simulink model "SRM"  (R2020a)
settings: Solver=VariableStepAuto  StartTime=0.0  StopTime=1  RelTol=1e-3
undefined symbols (not defined in the file): DiscIntNeverNeededParam, Ion, Lithium, Ts
libraries: powerlib x14, electricdrivelib x1
settings Model: Creator=Toan Thanh Nguyen  LastModifiedBy=NIKHIL
settings SFSimCC: CustomCodeUndefinedFunction=UseInterfaceOnly

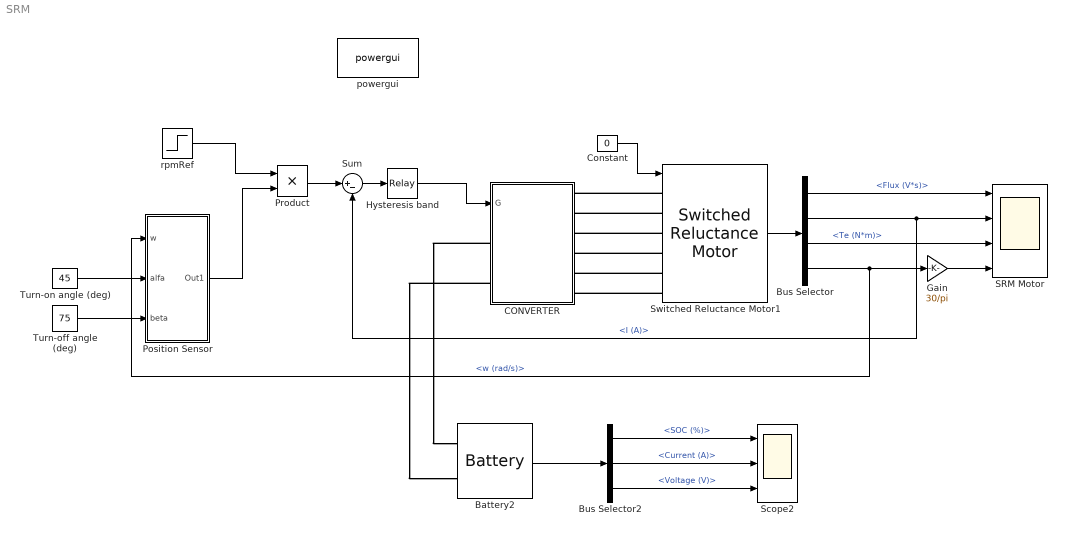
== system SRM ==
  Battery2 : electricdrivelib/Extra Sources/Battery  BatType=Lithium-Ion  ShowTempParam=off  ThermalPreset=no  ShowAgeParam=off  NomV=240  NomQ=5.4  SOC=100  Batt_Tr=30  PresetModel=on  MaxQ=5.4  MinV=180  FullV=279.3569  Dis_rate=2.3478  R=0.44444  Normal_OP=4.8835  expZone="[259.2926     0.2653043]"  current=[6.5 13 32.5]  Units=Time  Tci=20  NomT=20  T2=-30  MaxQ2=4.8  FullV2=7.1  Normal_OP2=5.655  expZone2="[6.58           1]"  Rca=0.6  ti=2000  Dp=0  Neq0=0  Tsim=1e6  Ta1=25  Qeol=5.4*0.9  Reol=0.013333*1.2  Char_age=[2.3478, 3]  Dis_age=[2.3478, 10]  N1=1500  N2=10500  N3=1000  N4=1400  Ta2=45  N5=950
  Bus Selector : BusSelector  OutputSignals=Flux (V*s),I (A),Te (N*m),w (rad/s)
  Bus Selector2 : BusSelector  OutputSignals=SOC (%),Current (A),Voltage (V)
  CONVERTER : Subsystem
  Constant : Constant  Value=0
  Gain : Gain  Gain=30/pi
  "Hysteresis band " : Relay  OnSwitchValue=10  OffSwitchValue=-10
  Position Sensor : Subsystem
  Product : Product
  SRM Motor : Scope  NumInputPorts=4
  Scope2 : Scope  NumInputPorts=3
  Sum : Sum  Inputs=|+-
  Switched Reluctance Motor1 : powerlib/Machines/Switched Reluctance Motor  MachineType=6/4  StatorResistance=0.05  Inertia=0.05  Friction=0.02  InitialSpeed=[0 0]  TsPowergui=0  TsBlock=Ts  MachineModel=Specific model  Lq=0.67e-3  Ld=23.6e-3  Lsat=0.15e-3  MaximumCurrent=450  MaximumFluxLinkage=0.486  Source=MAT-file  MagnetisationCharacteristic='srm64_60kw.mat'  RotorAngleVector=[0 10 20 30 40 45]  StatorCurrentVector=[0:25:450]  PlotCurves=off
      settings: SourceProductBaseCode=PS
  "Turn-off angle (deg) " : Constant  Value=75
  "Turn-on angle (deg) " : Constant  Value=45
  powergui : powerlib/powergui  Priority=1  SimulationMode=Discrete  SampleTime=1e-06  frequency=60  Iterations=50  frequencyindice=0  Pbase=100e6  ErrMax=1e-4  UnitsV=kV  UnitsW=MW  buscounter=0  FunctionMessages=off  echomessages=off  EnableUseOfTLC=off  CurrentSourceSwitches=off  DisableSnubberDevices=off  DisableRonSwitches=off  DisableVfSwitches=off  DisplayEquations=off  AutomaticDiscreteSolvers=off  SolverType=Tustin/Backward Euler (TBE)  Interpol=off  ExternalGateDelay=off  methode=off  Ts=100  x0status=blocks  SPID=on  SwTol=0  HookPort=off  NonlinearTolerance=0  nMaxIteration=15  ContinueOnMaxIteration=off  RestoreLinks=warning  ResistiveCurrentMeasurement=off  Frange=[0:2:500]  Ylog=off  Xlog=on  ShowGrid=off  save=off  variable=ZData  structure=0  ZoomFFT=off  StartTime=0.0  cycles=1  DisplayStyle=1  fundamental=60  FreqAxis=off  MaxFrequency=1000  frequencyindicesteady=1  RmsSteady=1  display=off
  rpmRef : Step  Time=0.1  Before=500  After=0  SampleTime=0
  wires:
  Constant/1 -> Switched Reluctance Motor1/1
  "Hysteresis band "/1 -> CONVERTER/1(G)
  Switched Reluctance Motor1/1 -> Bus Selector/1
  Bus Selector/4 -> Position Sensor/1(w), Gain/1  "<w (rad/s)>"
  Bus Selector/3 -> SRM Motor/3  "<Te (N*m)>"
  Bus Selector/2 -> Sum/2, SRM Motor/2  "<I (A)>"
  Bus Selector/1 -> SRM Motor/1  "<Flux (V*s)>"
  "Turn-on angle (deg) "/1 -> Position Sensor/2(alfa)
  "Turn-off angle (deg) "/1 -> Position Sensor/3(beta)
  Position Sensor/1(Out1) -> Product/2
  Product/1 -> Sum/1
  Sum/1 -> "Hysteresis band "/1
  Gain/1 -> SRM Motor/4
  rpmRef/1 -> Product/1
  Bus Selector2/2 -> Scope2/2  "<Current (A)>"
  Battery2/1 -> Bus Selector2/1
  Bus Selector2/1 -> Scope2/1  "<SOC (%)>"
  Bus Selector2/3 -> Scope2/3  "<Voltage (V)>"
  connections:
  Switched Reluctance Motor1/LConn6 -- CONVERTER/RConn6
  Switched Reluctance Motor1/LConn5 -- CONVERTER/RConn5
  Switched Reluctance Motor1/LConn4 -- CONVERTER/RConn4
  Switched Reluctance Motor1/LConn3 -- CONVERTER/RConn3
  Switched Reluctance Motor1/LConn2 -- CONVERTER/RConn2
  Switched Reluctance Motor1/LConn1 -- CONVERTER/RConn1
  CONVERTER/LConn1 -- Battery2/LConn1
  CONVERTER/LConn2 -- Battery2/LConn2

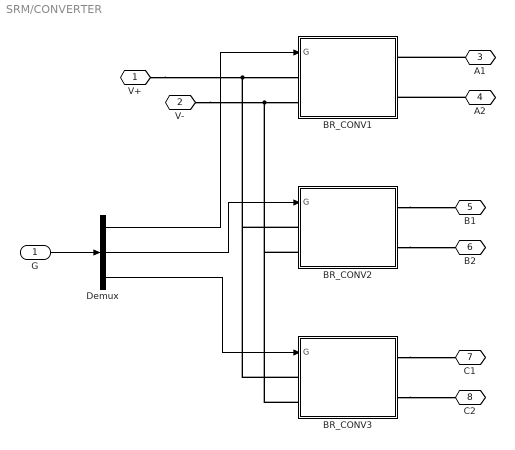
== system SRM/CONVERTER ==
  G : Inport
  BR_CONV1 : Subsystem
  BR_CONV2 : Subsystem
  BR_CONV3 : Subsystem
  Demux : Demux  Outputs=3
  V+ : PMIOPort  Side=Left
  V- : PMIOPort  Port=2  Side=Left
  A1 : PMIOPort  Port=3  Side=Right
  A2 : PMIOPort  Port=4  Side=Right
  B1 : PMIOPort  Port=5  Side=Right
  B2 : PMIOPort  Port=6  Side=Right
  C1 : PMIOPort  Port=7  Side=Right
  C2 : PMIOPort  Port=8  Side=Right
  wires:
  G/1 -> Demux/1
  Demux/1 -> BR_CONV1/1(G)
  Demux/2 -> BR_CONV2/1(G)
  Demux/3 -> BR_CONV3/1(G)
  connections:
  V-/RConn1 -- BR_CONV3/LConn2 -- BR_CONV2/LConn2 -- BR_CONV1/LConn2
  V+/RConn1 -- BR_CONV3/LConn1 -- BR_CONV2/LConn1 -- BR_CONV1/LConn1
  A1/RConn1 -- BR_CONV1/RConn1
  A2/RConn1 -- BR_CONV1/RConn2
  BR_CONV2/RConn1 -- B1/RConn1
  BR_CONV2/RConn2 -- B2/RConn1
  BR_CONV3/RConn1 -- C1/RConn1
  BR_CONV3/RConn2 -- C2/RConn1

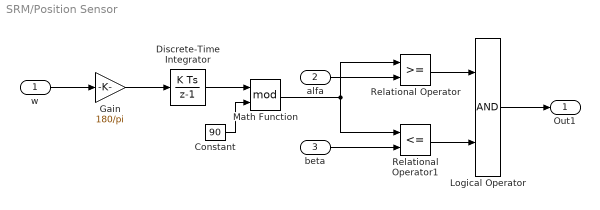
== system SRM/Position Sensor ==
  w : Inport
  alfa : Inport  Port=2
  beta : Inport  Port=3
  Constant : Constant  Value=90
  Discrete-Time Integrator : DiscreteIntegrator  InitialCondition=[0 -30 -60]  SampleTime=Ts  ICPrevOutput=DiscIntNeverNeededParam  ICPrevScaledInput=DiscIntNeverNeededParam
  Gain : Gain  Gain=180/pi
  Logical Operator : Logic  AllPortsSameDT=off  OutDataTypeStr=boolean
  Math Function : Math  Operator=mod  SignedPower=on  SaturateOnIntegerOverflow=on
  Relational Operator : RelationalOperator  OutDataTypeStr=boolean  RndMeth=Simplest
  Relational Operator1 : RelationalOperator  Operator=<=  OutDataTypeStr=boolean  RndMeth=Simplest
  Out1 : Outport  VectorParamsAs1DForOutWhenUnconnected=off
  wires:
  w/1 -> Gain/1
  Gain/1 -> Discrete-Time Integrator/1
  Discrete-Time Integrator/1 -> Math Function/1
  Constant/1 -> Math Function/2
  Math Function/1 -> Relational Operator/1, Relational Operator1/1
  alfa/1 -> Relational Operator/2
  beta/1 -> Relational Operator1/2
  Relational Operator/1 -> Logical Operator/1
  Relational Operator1/1 -> Logical Operator/2
  Logical Operator/1 -> Out1/1

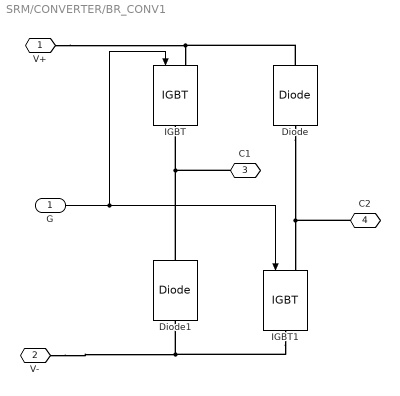
== system SRM/CONVERTER/BR_CONV1 ==
  G : Inport
  Diode : powerlib/Power Electronics/Diode  Ron=1E-3  Lon=0  Vf=0.8  IC=0  UseSnubber=0  Rs=1000  Cs=inf  Measurements=off
  Diode1 : powerlib/Power Electronics/Diode  Ron=1E-3  Lon=0  Vf=0.8  IC=0  UseSnubber=0  Rs=1000  Cs=inf  Measurements=off
  IGBT : powerlib/Power Electronics/IGBT  Ron=1E-3  Lon=0  Vf=1  Tf=1e-6  Tt=2e-6  IC=0  Rs=200  Cs=0.1E-06  Measurements=off
  IGBT1 : powerlib/Power Electronics/IGBT  Ron=1E-3  Lon=0  Vf=1  Tf=1e-6  Tt=2e-6  IC=0  Rs=200  Cs=0.1E-06  Measurements=off
  V+ : PMIOPort  Side=Left
  V- : PMIOPort  Port=2  Side=Left
  C1 : PMIOPort  Port=3  Side=Right
  C2 : PMIOPort  Port=4  Side=Right
  wires:
  G/1 -> IGBT1/1, IGBT/1
  connections:
  V+/RConn1 -- Diode/RConn1 -- IGBT/LConn1
  Diode/LConn1 -- C2/RConn1 -- IGBT1/LConn1
  IGBT1/RConn1 -- V-/RConn1 -- Diode1/LConn1
  Diode1/RConn1 -- C1/RConn1 -- IGBT/RConn1

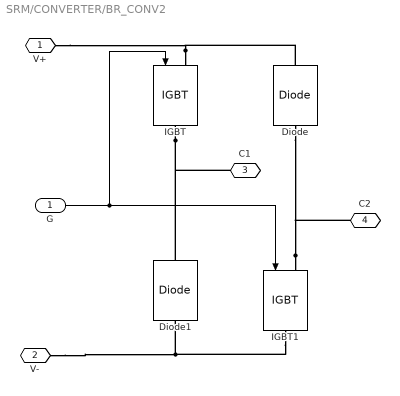
== system SRM/CONVERTER/BR_CONV2 ==
  G : Inport
  Diode : powerlib/Power Electronics/Diode  Ron=1E-3  Lon=0  Vf=0.8  IC=0  UseSnubber=0  Rs=1000  Cs=inf  Measurements=off
  Diode1 : powerlib/Power Electronics/Diode  Ron=1E-3  Lon=0  Vf=0.8  IC=0  UseSnubber=0  Rs=1000  Cs=inf  Measurements=off
  IGBT : powerlib/Power Electronics/IGBT  Ron=1E-3  Lon=0  Vf=1  Tf=1e-6  Tt=2e-6  IC=0  Rs=200  Cs=0.1E-06  Measurements=off
  IGBT1 : powerlib/Power Electronics/IGBT  Ron=1E-3  Lon=0  Vf=1  Tf=1e-6  Tt=2e-6  IC=0  Rs=200  Cs=0.1E-06  Measurements=off
  V+ : PMIOPort  Side=Left
  V- : PMIOPort  Port=2  Side=Left
  C1 : PMIOPort  Port=3  Side=Right
  C2 : PMIOPort  Port=4  Side=Right
  wires:
  G/1 -> IGBT1/1, IGBT/1
  connections:
  IGBT/LConn1 -- V+/RConn1 -- Diode/RConn1
  IGBT1/LConn1 -- Diode/LConn1 -- C2/RConn1
  IGBT1/RConn1 -- Diode1/LConn1 -- V-/RConn1
  IGBT/RConn1 -- Diode1/RConn1 -- C1/RConn1

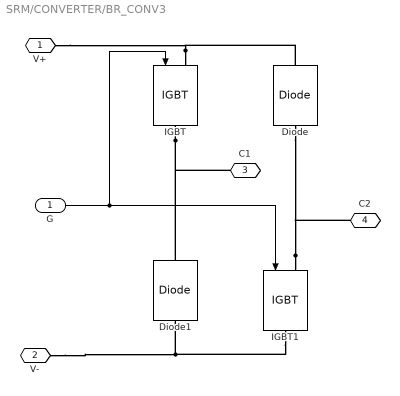
== system SRM/CONVERTER/BR_CONV3 ==
  G : Inport
  Diode : powerlib/Power Electronics/Diode  Ron=1E-3  Lon=0  Vf=0.8  IC=0  UseSnubber=0  Rs=1000  Cs=inf  Measurements=off
  Diode1 : powerlib/Power Electronics/Diode  Ron=1E-3  Lon=0  Vf=0.8  IC=0  UseSnubber=0  Rs=1000  Cs=inf  Measurements=off
  IGBT : powerlib/Power Electronics/IGBT  Ron=1E-3  Lon=0  Vf=1  Tf=1e-6  Tt=2e-6  IC=0  Rs=200  Cs=0.1E-06  Measurements=off
  IGBT1 : powerlib/Power Electronics/IGBT  Ron=1E-3  Lon=0  Vf=1  Tf=1e-6  Tt=2e-6  IC=0  Rs=200  Cs=0.1E-06  Measurements=off
  V+ : PMIOPort  Side=Left
  V- : PMIOPort  Port=2  Side=Left
  C1 : PMIOPort  Port=3  Side=Right
  C2 : PMIOPort  Port=4  Side=Right
  wires:
  G/1 -> IGBT1/1, IGBT/1
  connections:
  IGBT/LConn1 -- V+/RConn1 -- Diode/RConn1
  IGBT1/LConn1 -- Diode/LConn1 -- C2/RConn1
  IGBT1/RConn1 -- Diode1/LConn1 -- V-/RConn1
  IGBT/RConn1 -- Diode1/RConn1 -- C1/RConn1
